simulink model "BLDC_motor"  (R2020b)
settings: Solver=VariableStepAuto  StartTime=0.0  StopTime=10.0  RelTol=1e-3
model workspace (MAT data in the model file):
  B = 0.01
  J = 5
  KePhi = 1.6
  La = 0.1
  Ra = 0.5
  TL = 20
  Va = 160
  tau_a = 0.2
  tau_m = 500
libraries: powerlib x1
settings Model: Creator=mluser  LastModifiedBy=mluser

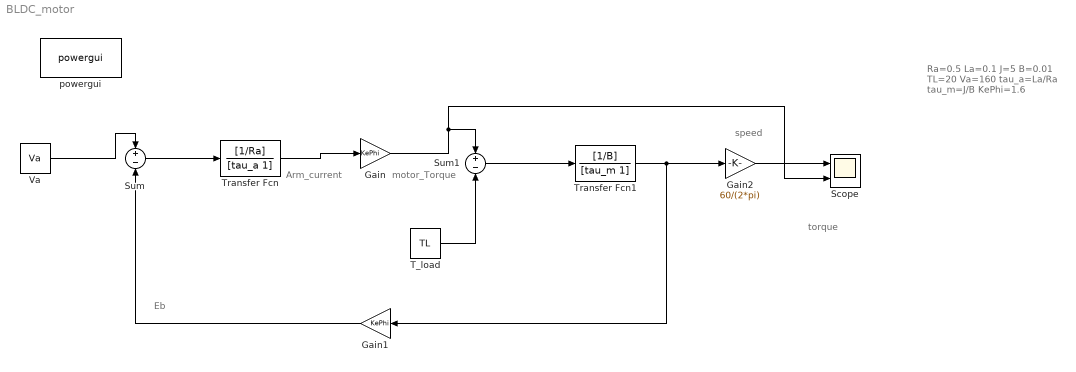
== system BLDC_motor ==
  note: Ra=0.5
      | La=0.1
      | J=5
      | B=0.01
      | TL=20
      | Va=160
      | tau_a=La/Ra
      | tau_m=J/B
      | KePhi=1.6
  note: torque
  note: speed
  note: Eb
  note: motor_Torque
  note: Arm_current
  Gain : Gain  Gain=KePhi
  Gain1 : Gain  Gain=KePhi
  Gain2 : Gain  Gain=60/(2*pi)
  Scope : Scope  NumInputPorts=2
  Sum : Sum  Inputs=+-
  Sum1 : Sum  Inputs=+-
  T_load : Constant  Value=TL
  Transfer Fcn : TransferFcn  Numerator=[1/Ra]  Denominator=[tau_a 1]
  Transfer Fcn1 : TransferFcn  Numerator=[1/B]  Denominator=[tau_m 1]
  Va : Constant  Value=Va
  powergui : powerlib/powergui  Priority=1  SimulationMode=Continuous  SampleTime=50e-6  frequency=60  Iterations=50  frequencyindice=60  Pbase=100e6  ErrMax=1e-4  UnitsV=kV  UnitsW=MW  buscounter=0  FunctionMessages=off  echomessages=off  EnableUseOfTLC=off  CurrentSourceSwitches=off  DisableSnubberDevices=off  DisableRonSwitches=off  DisableVfSwitches=off  DisplayEquations=off  AutomaticDiscreteSolvers=off  SolverType=Tustin/Backward Euler (TBE)  Interpol=off  ExternalGateDelay=off  methode=off  Ts=100  x0status=blocks  SPID=on  SwTol=0  HookPort=off  NonlinearTolerance=1e-4  nMaxIteration=100  ContinueOnMaxIteration=off  RestoreLinks=warning  ResistiveCurrentMeasurement=off  Frange=[0:2:500]  Ylog=off  Xlog=on  ShowGrid=off  save=off  variable=ZData  structure=0  ZoomFFT=off  StartTime=0.0  cycles=1  DisplayStyle=1  fundamental=60  FreqAxis=off  MaxFrequency=1000  frequencyindicesteady=1  RmsSteady=1  display=off
  wires:
  Va/1 -> Sum/1
  Sum/1 -> Transfer Fcn/1
  Transfer Fcn/1 -> Gain/1
  Gain/1 -> Scope/2, Sum1/1
  T_load/1 -> Sum1/2
  Sum1/1 -> Transfer Fcn1/1
  Transfer Fcn1/1 -> Gain1/1, Gain2/1
  Gain1/1 -> Sum/2
  Gain2/1 -> Scope/1
